simulink model "gm_hdl_modulator"  (R2017b)
settings: Solver=FixedStepDiscrete  StartTime=0.0  StopTime=10  RelTol=1e-3
libraries: simulink x1, hdlsllib x1
settings Model: Creator=jake  LastModifiedBy=mw
settings DataIOCC: SaveOutput=off  SaveTime=off
settings OptimizationCC: BlockReduction=off  ConditionallyExecuteInputs=off  DefaultParameterBehavior=Inlined
settings DebuggingCC: AlgebraicLoopMsg=error  InheritedTsInSrcMsg=none  SingleTaskRateTransMsg=error  StrictBusMsg=ErrorOnBusTreatedAsVector
settings HardwareCC: ProdBitPerPointer=32  ProdBitPerSizeT=32  ProdBitPerPtrDiffT=32  ProdLargestAtomicFloat=None  ProdIntDivRoundTo=Undefined  ProdEndianess=Unspecified  ProdWordSize=32  ProdHWDeviceType=ASIC/FPGA->ASIC/FPGA  ProdEqTarget=off
settings CodeAppCC: StateflowObjectComments=on
settings GRTTargetCC: TargetLangStandard=C89/C90 (ANSI)

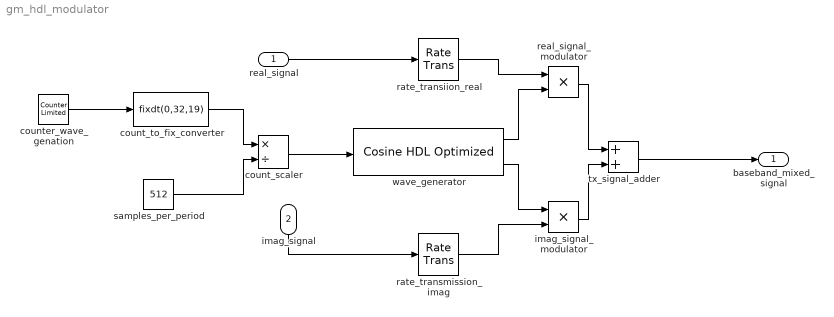
== system gm_hdl_modulator ==
  real_signal : Inport  OutDataTypeStr=fixdt(1, 20, 13)  PortDimensions=1  SampleTime=0.0001
  imag_signal : Inport  Port=2  OutDataTypeStr=fixdt(1, 20, 13)  PortDimensions=1  SampleTime=0.0001
  count_scaler : Product  Inputs=*/  OutMin=[0]  OutMax=[1]  OutDataTypeStr=fixdt(1,16)  SaturateOnIntegerOverflow=on  RndMeth=Zero
  count_to_fix_converter : DataTypeConversion  OutMin=[0]  OutMax=[511]  OutDataTypeStr=fixdt(0,32,19)
  counter_wave_genation : simulink/Sources/Counter Limited  uplimit=511  tsamp=1/10000
  imag_signal_modulator : Product
  rate_transiion_real : RateTransition
  rate_transmission_imag : RateTransition
  real_signal_modulator : Product
  samples_per_period : Constant  Value=512  OutDataTypeStr=fixdt(1,32,5)  SampleTime=-1
  tx_signal_adder : Sum
  wave_generator : hdlsllib/Lookup Tables/Cosine HDL Optimized  OutputFormula=sin(2*pi*u) and cos(2*pi*u)  NumDataPoints=512  TableDataTypeStr=fixdt(1,15,14)  SimulateLUTROMDelay=off
      settings: SourceProductName=HDL Coder  SourceProductBaseCode=HD
  baseband_mixed_signal : Outport  OutDataTypeStr=fixdt(1,37,27)  PortDimensions=[1 1]  SampleTime=[0.0001,0]
  wires:
  real_signal/1 -> rate_transiion_real/1
  imag_signal/1 -> rate_transmission_imag/1
  count_scaler/1 -> wave_generator/1
  count_to_fix_converter/1 -> count_scaler/1
  counter_wave_genation/1 -> count_to_fix_converter/1
  imag_signal_modulator/1 -> tx_signal_adder/2
  rate_transiion_real/1 -> real_signal_modulator/1
  rate_transmission_imag/1 -> imag_signal_modulator/2
  real_signal_modulator/1 -> tx_signal_adder/1
  samples_per_period/1 -> count_scaler/2
  tx_signal_adder/1 -> baseband_mixed_signal/1
  wave_generator/1 -> real_signal_modulator/2
  wave_generator/2 -> imag_signal_modulator/1
